simulink model "check_serial_new_arduino_basic"  (R2020b)
settings: Solver=FixedStepDiscrete  StartTime=0.0  StopTime=inf  FixedStep=0.1  RelTol=1e-3
undefined symbols (not defined in the file or in its folder): Serial_Port, Standard_Devices
libraries: sldrtlib x3
settings Model: Creator=Rahul Subramanian  LastModifiedBy=Rahul Subramanian

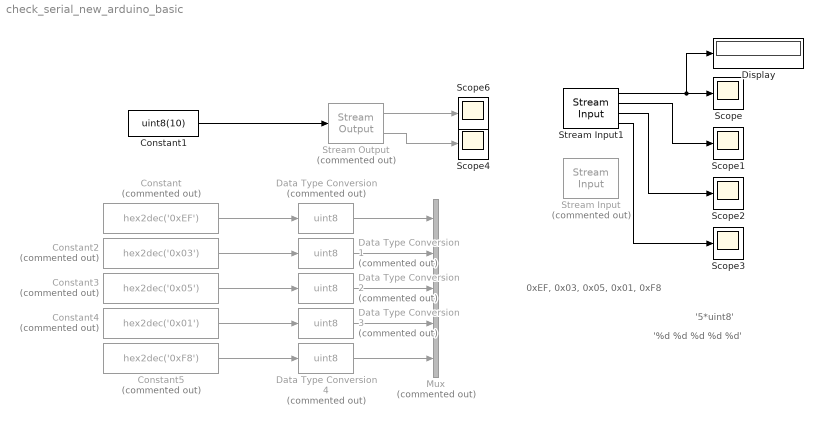
== system check_serial_new_arduino_basic ==
  note: '%d %d %d %d %d'
  note: '5*uint8'
  note: 0xEF, 0x03, 0x05, 0x01, 0xF8
  Constant : Constant  Commented=on  Value=hex2dec('0xEF')
  Constant1 : Constant  Value=uint8(10)
  Constant2 : Constant  Commented=on  Value=hex2dec('0x03')
  Constant3 : Constant  Commented=on  Value=hex2dec('0x05')
  Constant4 : Constant  Commented=on  Value=hex2dec('0x01')
  Constant5 : Constant  Commented=on  Value=hex2dec('0xF8')
  Data Type Conversion{,1..4} (5 alike) : DataTypeConversion  Commented=on  OutDataTypeStr=uint8
  Display : Display
  Mux : Mux  Commented=on  Inputs=5
  Scope{,1..4,6} (6 alike) : Scope
  Stream Input : sldrtlib/Stream Input  Commented=on  SampleTime=0.1  MaxMissedTicks=inf  ShowMissedTicks=on  YieldWhenWaiting=off  DrvName=Standard_Devices/Serial_Port  DrvAddress=5  DrvOptions=[19200 8 0 0 0 0 0 0]  DataTypes='5*uint8'  FormatString='%d%d%d%d%d'  Terminator={'\n'}  ShowReady=on  ShowError=on
      settings: AttributesFormatString=Serial Port [5]  SourceProductBaseCode=WT
  Stream Input1 : sldrtlib/Stream Input  SampleTime=0.1  MaxMissedTicks=inf  ShowMissedTicks=on  YieldWhenWaiting=off  DrvName=Standard_Devices/Serial_Port  DrvAddress=5  DrvOptions=[115200 8 0 0 0 0 0 0]  DataTypes='uint8'  FormatString='%d'  Terminator='\n'  ShowReady=on  ShowError=on
      settings: AttributesFormatString=Serial Port [5]  SourceProductBaseCode=WT
  Stream Output : sldrtlib/Stream Output  Commented=on  SampleTime=0.1  MaxMissedTicks=inf  ShowMissedTicks=off  YieldWhenWaiting=off  DrvName=Standard_Devices/Serial_Port  DrvAddress=5  DrvOptions=[115200 8 0 0 0 0 0 0]  PortSizes=[1]  FormatString='%d'  ShowReady=on  ShowError=on  InitialValue=[]  FinalValue=[]
      settings: AttributesFormatString=Serial Port [5]  SourceProductBaseCode=WT
  wires:
  Stream Input1/1 -> Display/1, Scope/1
  Stream Output/1 -> Scope6/1
  Stream Input1/2 -> Scope1/1
  Stream Input1/3 -> Scope2/1
  Stream Input1/4 -> Scope3/1
  Constant/1 -> Data Type Conversion/1
  Constant2/1 -> Data Type Conversion1/1
  Constant3/1 -> Data Type Conversion2/1
  Constant4/1 -> Data Type Conversion3/1
  Constant5/1 -> Data Type Conversion4/1
  Data Type Conversion/1 -> Mux/1
  Data Type Conversion1/1 -> Mux/2
  Data Type Conversion2/1 -> Mux/3
  Data Type Conversion3/1 -> Mux/4
  Data Type Conversion4/1 -> Mux/5
  Constant1/1 -> Stream Output/1
  Stream Output/2 -> Scope4/1
